simulink model "System_Template"  (R2021b)
settings: Solver=FixedStepDiscrete  StartTime=0.0  StopTime=0.001  RelTol=1e-3
model workspace (MAT data in the model file):
  test = 0
libraries: dsphdlxfrm x3, simulink x1, hdlsllib x1
settings Model: DataTypeOverride=Off  FPTShortcutValueString='{{},{''BaselineRun'',1,1,1,''BaselineRun'','''',{},''M'',''F'',''''},{''EmbeddedRun'',1,1,1,''EmbeddedRun'','''',{},''M'','''',''''}}'  Creator=max_d  LastModifiedBy=max_d
settings SolverCC: AlgebraicLoopSolver=TrustRegion  AutoInsertRateTranBlk=on
settings DataIOCC: LimitDataPoints=on  SaveOutput=off  SaveTime=off
settings OptimizationCC: BlockReduction=off  ConditionallyExecuteInputs=off  DefaultParameterBehavior=Inlined  InheritOutputTypeSmallerThanSingle=on  LifeSpan=inf
settings DebuggingCC: SignalRangeChecking=warning  AlgebraicLoopMsg=error  SingleTaskRateTransMsg=error  AllowSymbolicDim=off  StrictBusMsg=ErrorOnBusTreatedAsVector  SFUnexpectedBacktrackingDiag=warning  SFNoUnconditionalDefaultTransitionDiag=warning  SFExecutionAtInitializationDiag=none  SFMachineParentedDataDiag=warning  ArithmeticOperatorsInVariantConditions=warning
settings HardwareCC: ProdBitPerPointer=32  ProdBitPerSizeT=32  ProdBitPerPtrDiffT=32  ProdLargestAtomicFloat=None  ProdIntDivRoundTo=Undefined  ProdEndianess=Unspecified  ProdWordSize=32  ProdHWDeviceType=ASIC/FPGA->ASIC/FPGA  ProdEqTarget=off
settings SFSimCC: SimUseLocalCustomCode=off  CustomCodeUndefinedFunction=UseInterfaceOnly
settings RTWCC: RTWUseLocalCustomCode=off
settings CodeAppCC: StateflowObjectComments=on
settings GRTTargetCC: TargetLangStandard=C89/C90 (ANSI)
settings ConfigComp: CovScope=ReferencedModels  CovMetricSettings=dw  CovSaveCumulativeToWorkspaceVar=on  CovSaveSingleToWorkspaceVar=on  CovExternalEMLEnable=off  CovSFcnEnable=off

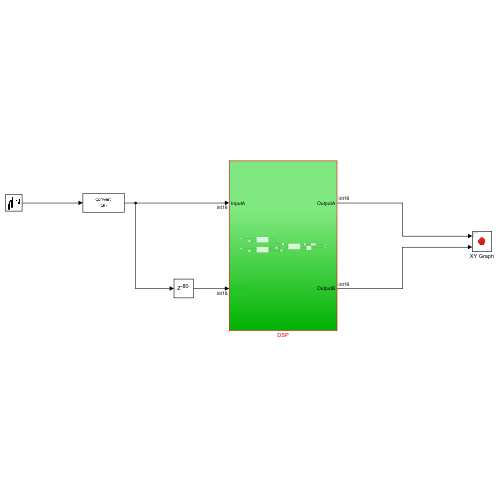
[thumbnail: Simulink's stored preview of the top-level diagram]
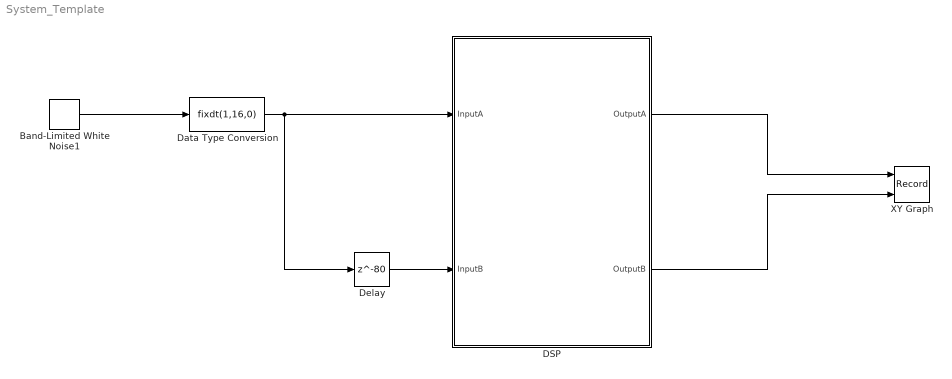
== system System_Template ==
  Band-Limited White Noise1 : simulink/Sources/Band-Limited White Noise  Cov=[0.1]  Ts=1/312.5e6  seed=[23341]
  DSP : Subsystem
  Data Type Conversion : DataTypeConversion  OutDataTypeStr=fixdt(1,16,0)  ConvertRealWorld=Stored Integer (SI)
  Delay : Delay  DelayLength=80  InitialCondition=0
  XY Graph : Record  FileSettingsInternal="{\"entries\":[{\"content\":{\"excelSettings\":{\"content\":{},\"type\":\"Streamout.ExcelSettings\"}},\"type\":\"Streamout.FileSettingStorage\",\"uuid\":\"6b793c2c-e135-4623-87cd-5f092496b2ec\"}],\"packageUris\":[\"http://schema.mathworks.com/mf0/streamout_blocks/R2020a\"],\"version\":\"1.0\"}"  Layout=[1 1]  SignalsInternal="{\"entries\":[{\"content\":{\"signals\":[{\"content\":{\"blockPath\":[\"System_Template/XY Graph\"],\"channel\":[],\"dimensions\":[1,1],\"domain\":\"System_Template/XY Graph\",\"lineColor\":\"#a2142f\",\"plots\":[1],\"port\":1,\"sid\":[\"\"],\"signalID\":29,\"signalName\":\"DSP:1\"},\"type\":\"RecordBlkView.Signal\",\"uuid\":\"2da7a736-7949-41f2-ad0b-a1a27dbd08a9\"},{\"content\":{\"blockPath\":[\"System_Template/XY Graph\"],\"channel\":[],\"dimensions\":[1],\"domain\":\"System_Template/XY Graph\",\"lineColor\":\"#139fff\",\"plots\":[1],\"port\":2,\"sid\":[\"\"],\"signalID\":33,\"signalName\":\"DSP:2\"},\"type\":\"RecordBlkView.Signal\",\"uuid\":\"2b468ea1-d406-416c-9993-6be0c50158d8\"}]},\"type\":\"RecordBlkView.InputSignals\",\"uuid\":\"ce3db894-6edc-4abb-9518-88b85b2ba208\"}],\"packageUris\":[\"http://schema.mathworks.com/mf0/streamout_blocks/R2020a\"],\"version\":\"1.0\"}"  VisualizationBindings="{\"xyplotplugin\":{\"info\":[{\"series\":[{\"bindingParametersList\":[{\"parameter\":\"X-Axis\",\"signalID\":33,\"signalName\":\"DSP:2\"},{\"parameter\":\"Y-Axis\",\"signalID\":29,\"signalName\":\"DSP:1\"}],\"seriesID\":57089}],\"subplotID\":1}]}}"  CompatibilityTag=XY
  wires:
  Band-Limited White Noise1/1 -> Data Type Conversion/1
  Delay/1 -> DSP/2(InputB)
  Data Type Conversion/1 -> Delay/1, DSP/1(InputA)
  DSP/2(OutputB) -> XY Graph/2
  DSP/1(OutputA) -> XY Graph/1

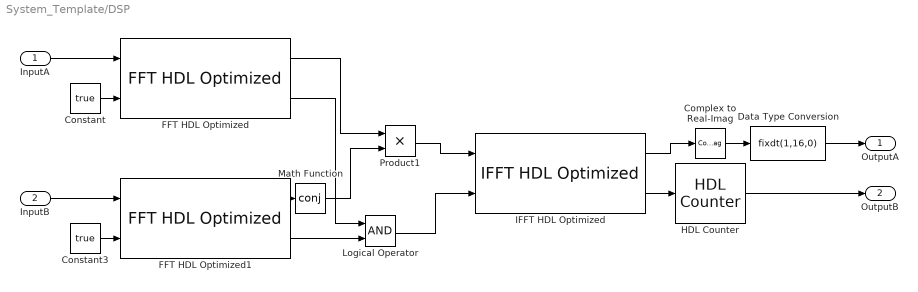
== system System_Template/DSP ==
  InputA : Inport  OutDataTypeStr=fixdt(1,16,0)
  InputB : Inport  Port=2  OutDataTypeStr=fixdt(1,16,0)
  Complex to Real-Imag : ComplexToRealImag  Output=Real
  Constant : Constant  Value=true  OutDataTypeStr=boolean  SampleTime=1/312.5e6
  Constant3 : Constant  Value=true  OutDataTypeStr=boolean  SampleTime=1/312.5e6
  Data Type Conversion : DataTypeConversion  OutDataTypeStr=fixdt(1,16,0)
  FFT HDL Optimized : dsphdlxfrm/FFT HDL Optimized  FFTLength=4096  Architecture=Streaming Radix 2^2  ComplexMultiplication=Use 4 multipliers and 2 adders  BitReversedOutput=on  BitReversedInput=off  Normalize=on  SimulateUsing=Code generation  RoundingMethod=Floor  ResetInputPort=off  StartOutputPort=off  EndOutputPort=off
      settings: SourceProductBaseCode=DS
  FFT HDL Optimized1 : dsphdlxfrm/FFT HDL Optimized  FFTLength=4096  Architecture=Streaming Radix 2^2  ComplexMultiplication=Use 4 multipliers and 2 adders  BitReversedOutput=on  BitReversedInput=off  Normalize=on  SimulateUsing=Code generation  RoundingMethod=Floor  ResetInputPort=off  StartOutputPort=off  EndOutputPort=off
      settings: SourceProductBaseCode=DS
  HDL Counter : hdlsllib/Sources/HDL Counter  CountType=Count limited  CountInit=4095  CountStep=-1  CountMax=0  CountFromType=Initial value  CountFrom=4095  CountResetPort=off  CountLoadPort=off  CountEnbPort=on  CountDirPort=off  CountHitOutputPort=off  CountDataType=Signed  CountWordLen=16  CountFracLen=0  CountSampTime=1
  IFFT HDL Optimized : dsphdlxfrm/IFFT HDL Optimized  FFTLength=4096  Architecture=Streaming Radix 2^2  ComplexMultiplication=Use 4 multipliers and 2 adders  BitReversedOutput=off  BitReversedInput=on  Normalize=on  SimulateUsing=Code generation  RoundingMethod=Floor  ResetInputPort=off  StartOutputPort=off  EndOutputPort=off
      settings: SourceProductBaseCode=DS
  Logical Operator : Logic  AllPortsSameDT=off  OutDataTypeStr=boolean
  Math Function : Math  Operator=conj  SaturateOnIntegerOverflow=on
  Product1 : Product
  OutputA : Outport  OutDataTypeStr=fixdt(1,16,0)  VectorParamsAs1DForOutWhenUnconnected=off
  OutputB : Outport  Port=2  OutDataTypeStr=fixdt(1,16,0)  VectorParamsAs1DForOutWhenUnconnected=off
  wires:
  Math Function/1 -> Product1/2
  IFFT HDL Optimized/2 -> HDL Counter/1
  Constant3/1 -> FFT HDL Optimized1/2
  Constant/1 -> FFT HDL Optimized/2
  FFT HDL Optimized/1 -> Product1/1
  Product1/1 -> IFFT HDL Optimized/1
  IFFT HDL Optimized/1 -> Complex to Real-Imag/1
  FFT HDL Optimized1/1 -> Math Function/1
  InputA/1 -> FFT HDL Optimized/1
  HDL Counter/1 -> OutputB/1
  InputB/1 -> FFT HDL Optimized1/1
  Complex to Real-Imag/1 -> Data Type Conversion/1
  Data Type Conversion/1 -> OutputA/1
  FFT HDL Optimized1/2 -> Logical Operator/2
  FFT HDL Optimized/2 -> Logical Operator/1
  Logical Operator/1 -> IFFT HDL Optimized/2
